simulink model "smc_plant"  (R2022a)
settings: Solver=VariableStepAuto  StartTime=0.0  StopTime=50  RelTol=1e-3
values from neighbouring files (symbols this model uses):
  d = 1.0    (= 1)    [init.m]
  kf1 = K2(1)    [init.m]
  kf2 = K2(2)    [init.m]
  ks = 0.02    [init.m]
  kv = 0.05    [init.m]
  M = 5    [init.m]
settings Model: Creator=Admin  LastModifiedBy=Admin

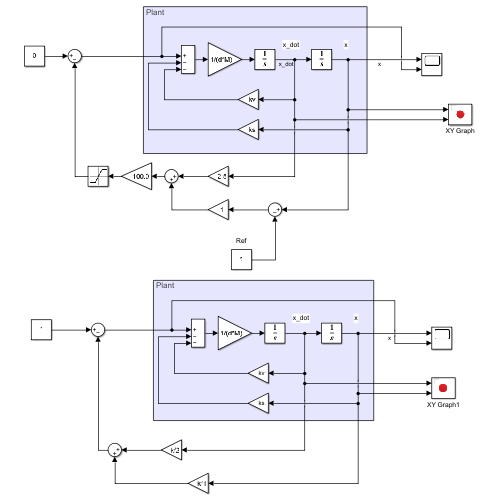
[thumbnail: Simulink's stored preview of the top-level diagram]
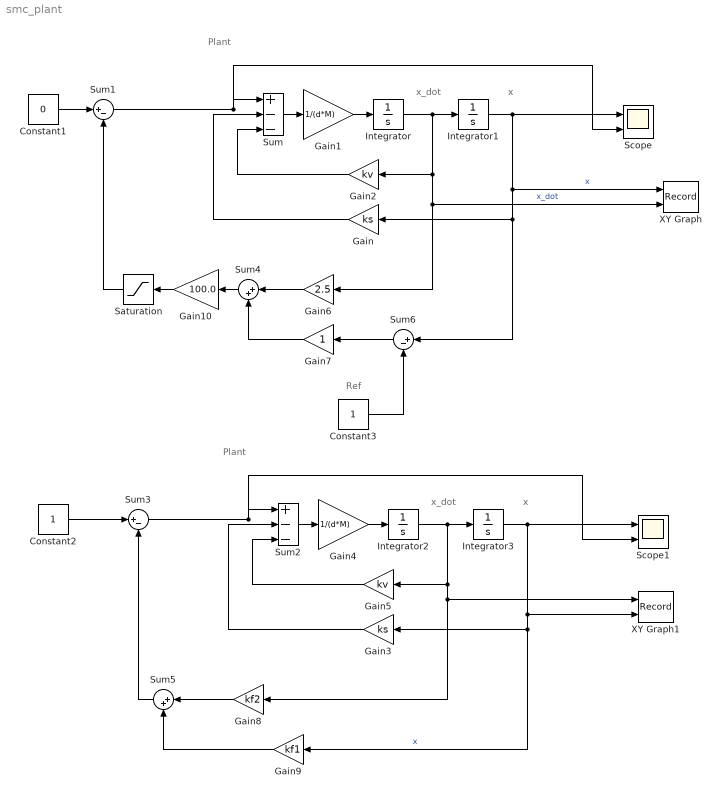
== system smc_plant ==
  note: Plant
  note: x
  note: x_dot
  note: Plant
  note: x_dot
  note: x
  note: Ref
  Constant1 : Constant  Value=0
  Constant2 : Constant
  Constant3 : Constant
  Gain : Gain  Gain=ks
  Gain1 : Gain  Gain=1/(d*M)
  Gain10 : Gain  Gain=100.0
  Gain2 : Gain  Gain=kv
  Gain3 : Gain  Gain=ks
  Gain4 : Gain  Gain=1/(d*M)
  Gain5 : Gain  Gain=kv
  Gain6 : Gain  Gain=2.5
  Gain7 : Gain
  Gain8 : Gain  Gain=kf2
  Gain9 : Gain  Gain=kf1
  Integrator{,1..3} (4 alike) : Integrator
  Saturation : Saturate  UpperLimit=1  LowerLimit=-1
  Scope : Scope  NumInputPorts=2
  Scope1 : Scope  NumInputPorts=2
  Sum : Sum  Inputs=|+--
  Sum1 : Sum  Inputs=|+-
  Sum2 : Sum  Inputs=|+--
  Sum3 : Sum  Inputs=|+-
  Sum4 : Sum  Inputs=|++
  Sum5 : Sum  Inputs=|++
  Sum6 : Sum  Inputs=|+-
  XY Graph : Record  FileSettingsInternal="{\"entries\":[{\"content\":{\"excelSettings\":{\"content\":{},\"type\":\"Streamout.ExcelSettings\"}},\"type\":\"Streamout.FileSettingStorage\",\"uuid\":\"edd0db5f-ca36-4a39-84dc-e90c1a7af110\"}],\"packageUris\":[\"http://schema.mathworks.com/mf0/streamout_blocks/R2020a\"],\"version\":\"1.0\"}"  Layout=[1 1]  SignalsInternal="{\"entries\":[{\"content\":{\"signals\":[{\"content\":{\"blockPath\":[\"smc_plant/XY Graph\"],\"channel\":[],\"dimensions\":[1],\"domain\":\"smc_plant/XY Graph\",\"lineColor\":\"#a2142f\",\"plots\":[1],\"port\":1,\"sid\":[\"\"],\"signalID\":832,\"signalName\":\"x\"},\"type\":\"RecordBlkView.Signal\",\"uuid\":\"91118d15-3883-49f9-8b8e-0d3cd413e352\"},{\"content\":{\"blockPath\":[\"smc_plant/XY Graph\"],\"channel\":[],\"dimensions\":[1],\"domain\":\"smc_plant/XY Graph\",\"lineColor\":\"#139fff\",\"plots\":[1],\"port\":2,\"sid\":[\"\"],\"signalID\":836,\"signalName\":\"x_dot\"},\"type\":\"RecordBlkView.Signal\",\"uuid\":\"ddb29860-e6ed-48e3-99fd-93dcf543f08b\"}]},\"type\":\"RecordBlkView.InputSignals\",\"uuid\":\"14719e05-0f5e-45ce-9b60-6b0442ad6763\"}],\"packageUris\":[\"http://schema.mathworks.com/mf0/streamout_blocks/R2020a\"],\"version\":\"1.0\"}"  VisualizationBindings="{\"xyplotplugin\":{\"info\":[{\"series\":[{\"bindingParametersList\":[{\"parameter\":\"X-Axis\",\"signalID\":832,\"signalName\":\"x\"},{\"parameter\":\"Y-Axis\",\"signalID\":836,\"signalName\":\"x_dot\"}],\"seriesID\":13084}],\"subplotID\":1}]}}"  CompatibilityTag=XY
  XY Graph1 : Record  FileSettingsInternal="{\"entries\":[{\"content\":{\"excelSettings\":{\"content\":{},\"type\":\"Streamout.ExcelSettings\"}},\"type\":\"Streamout.FileSettingStorage\",\"uuid\":\"8430d535-9f6d-4868-886c-4d4bacd11031\"}],\"packageUris\":[\"http://schema.mathworks.com/mf0/streamout_blocks/R2020a\"],\"version\":\"1.0\"}"  Layout=[1 1]  SignalsInternal="{\"entries\":[{\"content\":{\"signals\":[{\"content\":{\"blockPath\":[\"smc_plant/XY Graph1\"],\"channel\":[],\"dimensions\":[1],\"domain\":\"smc_plant/XY Graph1\",\"lineColor\":\"#a2142f\",\"plots\":[1],\"port\":1,\"sid\":[\"\"],\"signalID\":840,\"signalName\":\"Integrator2\"},\"type\":\"RecordBlkView.Signal\",\"uuid\":\"b8ee5012-be00-44fb-9010-90c6c5babbaf\"},{\"content\":{\"blockPath\":[\"smc_plant/XY Graph1\"],\"channel\":[],\"dimensions\":[1],\"domain\":\"smc_plant/XY Graph1\",\"lineColor\":\"#139fff\",\"plots\":[1],\"port\":2,\"sid\":[\"\"],\"signalID\":844,\"signalName\":\"x\"},\"type\":\"RecordBlkView.Signal\",\"uuid\":\"48915231-b629-4573-918f-7fdd75d20f22\"}]},\"type\":\"RecordBlkView.InputSignals\",\"uuid\":\"d1302127-25ba-43e7-9ba7-228bcb00bf33\"}],\"packageUris\":[\"http://schema.mathworks.com/mf0/streamout_blocks/R2020a\"],\"version\":\"1.0\"}"  VisualizationBindings="{\"xyplotplugin\":{\"info\":[{\"series\":[{\"bindingParametersList\":[{\"parameter\":\"X-Axis\",\"signalID\":840,\"signalName\":\"Integrator2\"},{\"parameter\":\"Y-Axis\",\"signalID\":844,\"signalName\":\"x\"}],\"seriesID\":19969}],\"subplotID\":1}]}}"  CompatibilityTag=XY
  wires:
  Integrator/1 -> XY Graph/2, Gain6/1, Gain2/1, Integrator1/1  "x_dot"
  Gain/1 -> Sum/2
  Integrator1/1 -> Scope/1, XY Graph/1, Sum6/1, Gain/1  "x"
  Sum/1 -> Gain1/1
  Gain1/1 -> Integrator/1
  Gain2/1 -> Sum/3
  Sum1/1 -> Scope/2, Sum/1
  Gain6/1 -> Sum4/1
  Gain7/1 -> Sum4/2
  Gain9/1 -> Sum5/2
  Sum3/1 -> Scope1/2, Sum2/1
  Constant2/1 -> Sum3/1
  Gain8/1 -> Sum5/1
  Sum5/1 -> Sum3/2
  Gain5/1 -> Sum2/3
  Sum2/1 -> Gain4/1
  Gain4/1 -> Integrator2/1
  Gain3/1 -> Sum2/2
  Integrator2/1 -> Gain8/1, XY Graph1/1, Gain5/1, Integrator3/1
  Integrator3/1 -> Scope1/1, XY Graph1/2, Gain9/1, Gain3/1  "x"
  Constant1/1 -> Sum1/1
  Sum6/1 -> Gain7/1
  Constant3/1 -> Sum6/2
  Saturation/1 -> Sum1/2
  Gain10/1 -> Saturation/1
  Sum4/1 -> Gain10/1
